simulink model "planarTether_th"  (R2018b)
settings: Solver=ode15s  StartTime=0.0  StopTime=sim_time  MaxStep=0.1  RelTol=1e-3  AbsTol=1e-3
values from neighbouring files (symbols this model uses):
  ini_length = sqrt(z_pos^2 + 2*amp^2)    [tester2.m]
  Vflow = [1;0]    [tester2.m]
libraries: planarTether_ul x1
settings Model: SimulationMode=accelerator  Creator=Ayaz  LastModifiedBy=Ayaz

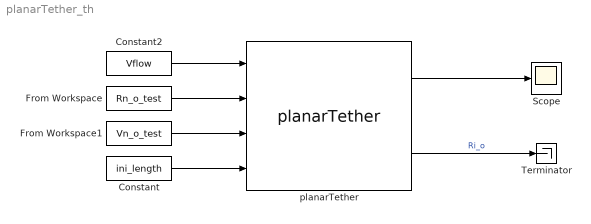
== system planarTether_th ==
  Constant : Constant  Value=ini_length  VectorParams1D=off
  Constant2 : Constant  Value=Vflow  VectorParams1D=off
  From Workspace : FromWorkspace  VariableName=Rn_o_test  SampleTime=0
  From Workspace1 : FromWorkspace  VariableName=Vn_o_test  SampleTime=0
  Scope : Scope
  Terminator : Terminator
  planarTether : planarTether_ul/planarTether  rhoF=rhoF  gravAcc=gravAcc  numNode=numNode  tetDia=tetDia  tetDensity=tetDensity  tetCD=Cd  tetYoungs=tetYoungs  tetZeta=tetYoungs  mT=mT
  wires:
  Constant2/1 -> planarTether/1
  From Workspace/1 -> planarTether/2
  From Workspace1/1 -> planarTether/3
  Constant/1 -> planarTether/4
  planarTether/1 -> Scope/1
  planarTether/2 -> Terminator/1  "Ri_o"
